simulink model "PMSM_modular_vector_control_sim"  (R2019a)
settings: Solver=ode4  StartTime=0.0  StopTime=Tfinal  FixedStep=Ts  RelTol=1e-3  EnableMultiTasking=on
values from neighbouring files (symbols this model uses):
  Cdc = 150e-6    (= 0.00015)    [PMSM_modular_vector_control_sim_parameters.m]    (also in PMSM_vector_control_single_parameters.m)
  IdPIDmax = Vdcm/5    (= 20)    [PMSM_modular_vector_control_sim_parameters.m]    (also in PMSM_vector_control_single_parameters.m = 54)
  IdPIDmin = -Vdcm/5    (= -20)    [PMSM_modular_vector_control_sim_parameters.m]    (also in PMSM_vector_control_single_parameters.m = -54)
  IdrefM1 = 0    [PMSM_modular_vector_control_sim_parameters.m]
  IdrefM2 = 0    [PMSM_modular_vector_control_sim_parameters.m]
  Inertia = 1e-2    (= 0.01)    [PMSM_modular_vector_control_sim_parameters.m]    (also in PMSM_vector_control_single_parameters.m)
  IqPIDmax = Vdcm-10    (= 90)    [PMSM_modular_vector_control_sim_parameters.m]    (also in PMSM_vector_control_single_parameters.m = 260)
  IqPIDmin = -(Vdcm-10)    (= -90)    [PMSM_modular_vector_control_sim_parameters.m]    (also in PMSM_vector_control_single_parameters.m = -260)
  IrefOverTref = MotorSpeedRad/(EfRated*3)    (= 0.261799387799)    [PMSM_modular_vector_control_sim_parameters.m]    (also in PMSM_vector_control_single_parameters.m)
  LoadTorque1 = 2    [PMSM_modular_vector_control_sim_parameters.m]    (also in PMSM_vector_control_single_parameters.m = 30)
  LoadTorque2 = 2    [PMSM_modular_vector_control_sim_parameters.m]    (also in PMSM_vector_control_single_parameters.m = 20)
  LoadTorqueStepTime = 3    [PMSM_modular_vector_control_sim_parameters.m]    (also in PMSM_vector_control_single_parameters.m = 0.5)
  MechanicalLoadTorque1 = 2    [PMSM_modular_vector_control_sim_parameters.m]
  phase = [0 0 0 0]    [PMSM_modular_vector_control_sim_parameters.m]    (also in PMSM_vector_control_single_parameters.m)
  PMSMLoadResistance = 1e3    (= 1000)    [PMSM_modular_vector_control_sim_parameters.m]
  PolePairs = 10    [PMSM_modular_vector_control_sim_parameters.m]    (also in PMSM_vector_control_single_parameters.m)
  Rin = 1e-3    (= 0.001)    [PMSM_modular_vector_control_sim_parameters.m]    (also in PMSM_vector_control_single_parameters.m)
  Ripth = 0.1    [PMSM_modular_vector_control_sim_parameters.m]    (also in PMSM_vector_control_single_parameters.m)
  Rs = 321e-3    (= 0.321)    [PMSM_modular_vector_control_sim_parameters.m]    (also in PMSM_vector_control_single_parameters.m)
  SpeedPIDmax = 20    [PMSM_modular_vector_control_sim_parameters.m]    (also in PMSM_vector_control_single_parameters.m = 60)
  SpeedPIDmin = -20    [PMSM_modular_vector_control_sim_parameters.m]    (also in PMSM_vector_control_single_parameters.m = -60)
  SpeedRef1 = 200    [PMSM_modular_vector_control_sim_parameters.m]    (also in PMSM_vector_control_single_parameters.m = 600)
  SpeedRef2 = 100    [PMSM_modular_vector_control_sim_parameters.m]    (also in PMSM_vector_control_single_parameters.m = 200)
  SpeedRefStepTime = 6    [PMSM_modular_vector_control_sim_parameters.m]    (also in PMSM_vector_control_single_parameters.m = 0.5)
  Ts = 1000e-9    (= 1e-06)    [PMSM_modular_vector_control_sim_parameters.m]    (also in PMSM_vector_control_single_parameters.m)
  Vdc = 200    [PMSM_modular_vector_control_sim_parameters.m]    (also in PMSM_vector_control_single_parameters.m = 270)
  Vin = Vdc + Rin*(Pout/Vdc)    (= 200.01)    [PMSM_modular_vector_control_sim_parameters.m]    (also in PMSM_vector_control_single_parameters.m = 270.007407407)
  ViscousFriction = 1e-3    (= 0.001)    [PMSM_modular_vector_control_sim_parameters.m]    (also in PMSM_vector_control_single_parameters.m)
undefined symbols (not defined in the file or in its folder): Lload, Rload
libraries: powerlib x41, powerlib_meascontrol x33, fl_lib x12, simulink x9, nesl_utility x8, sdl_lib x2
(part 1 of 2)
settings Model: Creator=ugurm  LastModifiedBy=hakan
settings DataIOCC: LimitDataPoints=on  SaveFormat=Array  ReturnWorkspaceOutputs=off
settings OptimizationCC: LifeSpan=inf
settings DebuggingCC: UnderspecifiedInitializationDetection=Classic  MergeDetectMultiDrivingBlocksExec=none  SolverPrmCheckMsg=warning  StateNameClashWarn=warning  SFUnexpectedBacktrackingDiag=warning  SFNoUnconditionalDefaultTransitionDiag=warning  ArithmeticOperatorsInVariantConditions=warning
settings HardwareCC: ProdBitPerPointer=32  ProdBitPerSizeT=32  ProdBitPerPtrDiffT=32  ProdLargestAtomicFloat=None  ProdIntDivRoundTo=Undefined  ProdEndianess=Unspecified  ProdWordSize=32  ProdHWDeviceType=32-bit Generic
settings ModelReferenceCC: PropagateSignalLabelsOutOfModel=off
settings SFSimCC: SimUseLocalCustomCode=off
settings RTWCC: RTWUseLocalCustomCode=off
settings CodeAppCC: StateflowObjectComments=on
settings GRTTargetCC: TargetLangStandard=C89/C90 (ANSI)  GeneratePreprocessorConditionals=Disable all
settings ConfigComp: CovMetricSettings=dw  CovHtmlReporting=on  CovSaveCumulativeToWorkspaceVar=on  CovSaveSingleToWorkspaceVar=on  CovExternalEMLEnable=off
settings SimscapeCC: SimscapeNormalizeSystem=off

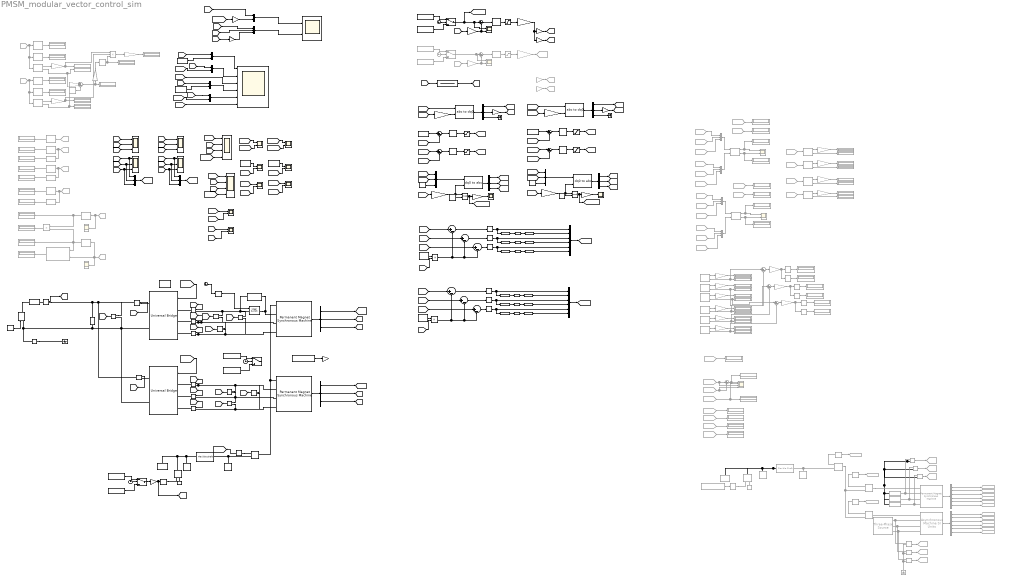
== system PMSM_modular_vector_control_sim ==
  Asynchronous Machine SI Units2 : powerlib/Machines/Asynchronous Machine SI Units  Commented=on  RotorType=Squirrel-cage  PresetModel="16:  10 HP (7.5KW)  400 V 50Hz 1440 RPM"  MechanicalLoad=Mechanical rotational port  ShowDetailedParameters=on  ReferenceFrame=Rotor  Units=SI  MeasurementBus=off  NominalParameters=[7500 400 50]  Stator=[0.7384 0.003045]  Rotor=[0.7402 0.003045]  Cage1=[0.4155 0.002066]  Cage2=[0.4168 0.0003495]  Lm=0.1241  Mechanical=[0.0343 0.000503 2]  PolePairs=2  InitialConditions=[0 0 0 0 0 0 0 0]  SimulateSaturation=off  Saturation=[14.03593122, 27.81365428, 53.79336849, 72.68890987, 97.98006896, 148.6815601, 215.7428561, 302.9841135, 428.7778367 ; 230, 322, 414, 460, 506, 552, 598, 644, 690]  LoadFlowParameters=1492000  TsPowergui=0  TsBlock=-1  IterativeModel=Trapezoidal non iterative  IterativeDiscreteModel=Trapezoidal non iterative  Pmec=1.492e+006
      settings: SourceProductName=Simscape Electrical
  Bus Creator : BusCreator  Inputs=3
  Bus Creator{1..5} (5 alike) : BusCreator  Inputs=2
  Bus Selector : BusSelector  Commented=on  OutputSignals=Mechanical.Rotor speed (wm),Mechanical.Electromagnetic torque Te (N*m),Mechanical.Rotor angle thetam (rad),Stator measurements.Stator current is_a (A),Stator measurements.Stator current is_b (A),Stator measurements.Stator current is_c (A)
  Bus Selector1 : BusSelector  Commented=on  OutputSignals=Rotor speed wm (rad/s),Electromagnetic torque Te (N*m),Rotor angle thetam (rad),Stator current is_a (A),Stator current is_b (A),Stator current is_c (A)
  Bus Selector2 : BusSelector  OutputSignals=Rotor angle thetam (rad),Rotor speed wm (rad/s),Electromagnetic torque Te (N*m)
  Bus Selector3 : BusSelector  OutputSignals=Rotor angle thetam (rad),Rotor speed wm (rad/s),Electromagnetic torque Te (N*m)
  Clock{,1..2,4} (4 alike) : Clock
  Clock3 : Clock  Commented=on
  Compare To Constant : simulink/Logic and Bit Operations/Compare To Constant  relop=<=  const=3.0  OutDataTypeStr=boolean
  Constant1 : Constant  Value=Vin
  Constant10 : Constant  Value=2*pi
  Constant11 : Constant  Value=SpeedRef2
  Constant13 : Constant  Value=LoadTorque2
  Constant16 : Constant  Value=LoadTorque1
  Constant17 : Constant  Commented=on  Value=SpeedRef2
  Constant18 : Constant  Commented=on  Value=SpeedRef1
  Constant19 : Constant  Value=LoadTorque2
  Constant20 : Constant  Value=LoadTorque1
  Constant3 : Constant  Commented=on  Value=-MechanicalLoadTorque1
  Constant4 : Constant  Value=MechanicalLoadTorque1
  Constant5 : Constant  Value=2*pi
  Constant6 : Constant  Value=SpeedRef1
  Constant7 : Constant  Value=0
  Constant8 : Constant  Value=0
  Constant9 : Constant  Commented=on  Value=sqrt(3)
  Current Measurement : powerlib/Measurements/Current Measurement  PhasorSimulation=off  OutputType=Complex  PSBequivalent=0
      settings: SourceProductName=Simscape Electrical
  Current Measurement1 : powerlib/Measurements/Current Measurement  PhasorSimulation=off  OutputType=Complex  PSBequivalent=0
      settings: SourceProductName=Simscape Electrical
  Data Type Conversion{1,3,5,7,9,11} (6 alike) : DataTypeConversion  OutDataTypeStr=boolean
  Data Type Conversion{2,4,6,8,10,12} (6 alike) : DataTypeConversion  OutDataTypeStr=double
  Demux{,1..3} (4 alike) : Demux  Outputs=3
  Display{,1..62} (63 alike) : Display  Commented=on
  Flexible Shaft : sdl_lib/Couplings & Drives/Flexible Shaft  Commented=on  modelTransverse=simscape.enum.onoff.off  parameterization=1  n_segments=10  shaft_stiffness=MechanicalShaftStiffness N*m/rad  shaft_inertia=MechanicalShaftInertia kg*m^2  length=1 m  eiIN=5e5 m^4*Pa  rhoaIN=19 kg/m  shaft_construction=1  diameter_outer=0.075 m  diameter_inner=0.05 m  density=7.8e+3 kg/m^3  shear_modulus=7.93e+10 Pa  elastic_modulus=200e9 Pa  damping_ratio=MechanicalShaftDampingRatio  mu_visc=[ 0 0 ] N*m/(rad/s)  boundaryC=sdl.enum.shaftSupport.clamp  KtransC_row=[10000000, 10000000] N/m  KrotC_row=[10000000, 10000000] N*m/rad  boundaryR=sdl.enum.shaftSupport.clamp  KtransR_row=[10000000, 10000000] N/m  KrotR_row=[10000000, 10000000] N*m/rad  alpha=10 1/s  beta=1e-8 s  d_bearing_trans=[0, 0] N/(m/s)  d_bearing_rotation=[0, 0] N*m/(rad/s)  noDisk=sdl.enum.shaftDisks.none  zDisk=0.5 m  mDiskIN=2 kg  IdDiskIN=0.025 kg*m^2  IpDiskIN=0.050 kg*m^2  offsetMR=[.01, .01] m*kg  offsetMassLocation=[.33, .67] m  offsetMR_initialAngleIN=[0, pi] rad  AnalysisMethod=sdl.enum.bendingAnalysisMethod.LumpedMass  ModeInputMethod=sdl.enum.modeInputMethod.SimscapeDetermined  numModesIn=6  OmegaNom=100 rpm  dw=5 rad/s  dwRefineFactor=1e-4  wMax=50000 rad/s  dz=0.01 m  userMode_w=[162, 162, 649, 649, 1460, 1460, 2596, 2596] rad/s  userMode_z=[0 : 0.1 : 1] m  userMode_shape=[0, 0, 0, 0, 0, 0, 0, 0, 0, 0, 0, 0, 0, 0, 0, 0; .309, 0, 0, .309, .5878, 0, 0, .5878, .809, 0, 0, .809, .9511, 0, 0, .9511; .5878, 0, 0, .5878, .9511, 0, 0, .9511, .9511, 0, 0, .9511, .5878, 0, 0, .5878; .809, 0, 0, .809, .9511, 0, 0, .9511, .309, 0, 0, .309, -.5878, 0, 0, -.5878; .9511, 0, 0, .9511, .5878, 0, 0, .5878, -.5878, 0, 0, -.5878, -.9511, 0, 0, -.9511; 1, 0, 0, 1, 0, 0, 0, 0, -1, 0, 0, -1, 0, 0, 0, 0; .9511, 0, 0, .9511, -.5878, 0, 0, -.5878, -.5878, 0, 0, -.5878, .9511, 0, 0, .9511; .809, 0, 0, .809, -.9511, 0, 0, -.9511, .309, 0, 0, .309, .5878, 0, 0, .5878; .5878, 0, 0, .5878, -.9511, 0, 0, -.9511, .9511, 0, 0, .9511, -.5878, 0, 0, -.5878; .309, 0, 0, .309, -.5878, 0, 0, -.5878, .809, 0, 0, .809, -.9511, 0, 0, -.9511; 0, 0, 0, 0, 0, 0, 0, 0, 0, 0, 0, 0, 0, 0, 0, 0]  initial_deflection=0 rad  initial_velocity=0 rpm
      settings: SourceProductName=Simscape Driveline  SourceProductBaseCode=LD
  Flexible Shaft1 : sdl_lib/Couplings & Drives/Flexible Shaft  modelTransverse=simscape.enum.onoff.off  parameterization=1  n_segments=10  shaft_stiffness=MechanicalShaftStiffness N*m/rad  shaft_inertia=MechanicalShaftInertia kg*m^2  length=1 m  eiIN=5e5 m^4*Pa  rhoaIN=19 kg/m  shaft_construction=1  diameter_outer=0.075 m  diameter_inner=0.05 m  density=7.8e+3 kg/m^3  shear_modulus=7.93e+10 Pa  elastic_modulus=200e9 Pa  damping_ratio=MechanicalShaftDampingRatio  mu_visc=[ 0 0 ] N*m/(rad/s)  boundaryC=sdl.enum.shaftSupport.clamp  KtransC_row=[10000000, 10000000] N/m  KrotC_row=[10000000, 10000000] N*m/rad  boundaryR=sdl.enum.shaftSupport.clamp  KtransR_row=[10000000, 10000000] N/m  KrotR_row=[10000000, 10000000] N*m/rad  alpha=10 1/s  beta=1e-8 s  d_bearing_trans=[0, 0] N/(m/s)  d_bearing_rotation=[0, 0] N*m/(rad/s)  noDisk=sdl.enum.shaftDisks.none  zDisk=0.5 m  mDiskIN=2 kg  IdDiskIN=0.025 kg*m^2  IpDiskIN=0.050 kg*m^2  offsetMR=[.01, .01] m*kg  offsetMassLocation=[.33, .67] m  offsetMR_initialAngleIN=[0, pi] rad  AnalysisMethod=sdl.enum.bendingAnalysisMethod.LumpedMass  ModeInputMethod=sdl.enum.modeInputMethod.SimscapeDetermined  numModesIn=6  OmegaNom=100 rpm  dw=5 rad/s  dwRefineFactor=1e-4  wMax=50000 rad/s  dz=0.01 m  userMode_w=[162, 162, 649, 649, 1460, 1460, 2596, 2596] rad/s  userMode_z=[0 : 0.1 : 1] m  userMode_shape=[0, 0, 0, 0, 0, 0, 0, 0, 0, 0, 0, 0, 0, 0, 0, 0; .309, 0, 0, .309, .5878, 0, 0, .5878, .809, 0, 0, .809, .9511, 0, 0, .9511; .5878, 0, 0, .5878, .9511, 0, 0, .9511, .9511, 0, 0, .9511, .5878, 0, 0, .5878; .809, 0, 0, .809, .9511, 0, 0, .9511, .309, 0, 0, .309, -.5878, 0, 0, -.5878; .9511, 0, 0, .9511, .5878, 0, 0, .5878, -.5878, 0, 0, -.5878, -.9511, 0, 0, -.9511; 1, 0, 0, 1, 0, 0, 0, 0, -1, 0, 0, -1, 0, 0, 0, 0; .9511, 0, 0, .9511, -.5878, 0, 0, -.5878, -.5878, 0, 0, -.5878, .9511, 0, 0, .9511; .809, 0, 0, .809, -.9511, 0, 0, -.9511, .309, 0, 0, .309, .5878, 0, 0, .5878; .5878, 0, 0, .5878, -.9511, 0, 0, -.9511, .9511, 0, 0, .9511, -.5878, 0, 0, -.5878; .309, 0, 0, .309, -.5878, 0, 0, -.5878, .809, 0, 0, .809, -.9511, 0, 0, -.9511; 0, 0, 0, 0, 0, 0, 0, 0, 0, 0, 0, 0, 0, 0, 0, 0]  initial_deflection=0 rad  initial_velocity=0 rpm
      settings: SourceProductName=Simscape Driveline  SourceProductBaseCode=LD
  Fourier1 : powerlib_meascontrol/Measurements/Fourier  Commented=on  Freq=fout  n=1  InInit=[0, 0]  Ts=Ts
      settings: SourceProductName=Simscape Electrical
  Fourier10 : powerlib_meascontrol/Measurements/Fourier  Commented=on  Freq=100  n=1  InInit=[0, 0]  Ts=0
      settings: SourceProductName=Simscape Electrical
  Fourier{3..8,11..12} (8 alike) : powerlib_meascontrol/Measurements/Fourier  Commented=on  Freq=50  n=1  InInit=[0, 0]  Ts=0
      settings: SourceProductName=Simscape Electrical
  Fourier2 : powerlib_meascontrol/Measurements/Fourier  Commented=on  Freq=fout  n=1  InInit=[0, 0]  Ts=Ts
      settings: SourceProductName=Simscape Electrical
  Fourier9 : powerlib_meascontrol/Measurements/Fourier  Commented=on  Freq=100  n=1  InInit=[0, 0]  Ts=0
      settings: SourceProductName=Simscape Electrical
  From : From  Commented=on  GotoTag=Vdc
  From1 : From  Commented=on  GotoTag=Iin
  From12 : From  Commented=on  GotoTag=Isa
  From15 : From  Commented=on  GotoTag=Vab
  From2 : From  Commented=on  GotoTag=Iin
  From3 : From  Commented=on  GotoTag=Idc2
  From30 : From  Commented=on  GotoTag=TorqueM1
  From31 : From  Commented=on  GotoTag=SpeedM1
  From32 : From  Commented=on  GotoTag=TorqueM2
  From33 : From  Commented=on  GotoTag=TorqueM2
  From34 : From  Commented=on  GotoTag=VM2PhA
  From35 : From  Commented=on  GotoTag=TorqueTotal
  From36 : From  Commented=on  GotoTag=TorqueMod1
  From37 : From  Commented=on  GotoTag=TorqueMod2
  From38 : From  Commented=on  GotoTag=TorqueM1
  From39 : From  Commented=on  GotoTag=TorqueM1
  From4 : From  Commented=on  GotoTag=Icap
  From40 : From  Commented=on  GotoTag=VM1PhA
  From41 : From  Commented=on  GotoTag=VM1PhB
  From42 : From  Commented=on  GotoTag=VM1PhC
  From43 : From  Commented=on  GotoTag=IM1PhA
  From44 : From  Commented=on  GotoTag=IM1PhB
  From45 : From  Commented=on  GotoTag=IM1PhC
  From46 : From  Commented=on  GotoTag=VM2PhB
  From47 : From  Commented=on  GotoTag=VM2PhC
  From48 : From  Commented=on  GotoTag=IM2PhA
  From49 : From  Commented=on  GotoTag=IM2PhB
  From5 : From  Commented=on  GotoTag=SpeedM1
  From50 : From  Commented=on  GotoTag=IM2PhC
  From51 : From  Commented=on  GotoTag=SpeedM2
  From52 : From  Commented=on  GotoTag=TorqueM2
  From53 : From  Commented=on  GotoTag=VM1PhA
  From54 : From  Commented=on  GotoTag=IM1PhA
  From55 : From  Commented=on  GotoTag=VM2PhA
  From56 : From  Commented=on  GotoTag=IM2PhA
  From58 : From  Commented=on  GotoTag=Idc1
  From92 : From  Commented=on  GotoTag=wmM2
  Gain{,4,26,28} (4 alike) : Gain  Gain=PolePairs
  Gain{1,9,13..22} (12 alike) : Gain  Commented=on  Gain=1/sqrt(2)
  Gain{6,8,10,12} (4 alike) : Gain  Commented=on  Gain=pi/180
  Gain11 : Gain
  Gain2 : Gain  Gain=30/pi
  Gain23 : Gain  Gain=0.5
  Gain24 : Gain  Gain=0.5
  Gain25 : Gain  Gain=0.5
  Gain27 : Gain
  Gain29 : Gain  Gain=180/pi
  Gain3 : Gain  Gain=IrefOverTref
  Gain30 : Gain  Commented=on  Gain=30/pi
  Gain31 : Gain  Commented=on  Gain=0.5
  Gain32 : Gain  Commented=on  Gain=0.5
  Gain33 : Gain  Commented=on  Gain=IrefOverTref
  Gain34 : Gain  Gain=-2
  Gain35 : Gain  Gain=1/PolePairs
  Gain36 : Gain  Gain=-1
  Gain5 : Gain  Commented=on  Gain=sqrt(3)
  Gain7 : Gain  Gain=180/pi
  Goto2 : Goto  Commented=on  GotoTag=IqrefM2
  Goto24 : Goto  Commented=on  GotoTag=ThetaM2
  Goto25 : Goto  Commented=on  GotoTag=TorqueM2
  Goto26 : Goto  Commented=on  GotoTag=SpeedM2
  Goto27 : Goto  Commented=on  GotoTag=ThetaM1
  Goto28 : Goto  Commented=on  GotoTag=TorqueM1
  Goto29 : Goto  Commented=on  GotoTag=SpeedM1
  Goto30 : Goto  Commented=on  GotoTag=TorqueTotal
  Goto31 : Goto  Commented=on  GotoTag=TorqueMod1
  Goto32 : Goto  Commented=on  GotoTag=TorqueMod2
  Goto33 : Goto  Commented=on  GotoTag=VM1PhA
  Goto34 : Goto  Commented=on  GotoTag=VM1PhB
  Goto35 : Goto  Commented=on  GotoTag=VM1PhC
  Goto36 : Goto  Commented=on  GotoTag=IM1PhC
  Goto37 : Goto  Commented=on  GotoTag=IM1PhB
  Goto38 : Goto  Commented=on  GotoTag=IM1PhA
  Goto39 : Goto  Commented=on  GotoTag=IM2PhC
  Goto40 : Goto  Commented=on  GotoTag=IM2PhB
  Goto41 : Goto  Commented=on  GotoTag=IM2PhA
  Goto42 : Goto  Commented=on  GotoTag=VM2PhA
  Goto43 : Goto  Commented=on  GotoTag=VM2PhB
  Goto44 : Goto  Commented=on  GotoTag=VM2PhC
  Goto69 : Goto  Commented=on  GotoTag=IqrefM1
  Goto70 : Goto  Commented=on  GotoTag=IqrefM2
  Ground1 : powerlib/Elements/Ground  Commented=on  LConnTagsString=a
      settings: SourceProductName=Simscape Electrical
  Ground5 : powerlib/Elements/Ground  LConnTagsString=a
      settings: SourceProductName=Simscape Electrical
  Idc_m{1,3..5,14,16..17} (7 alike) : powerlib/Measurements/Current Measurement  PhasorSimulation=off  OutputType=Complex  PSBequivalent=0
      settings: SourceProductName=Simscape Electrical
  Ideal Switch : powerlib/Power Electronics/Ideal Switch  Ron=0.001  Lon=0  IC=0  Rs=1e5  Cs=inf  Measurements=on
      settings: SourceProductName=Simscape Electrical
  Ideal Torque Sensor1 : fl_lib/Mechanical/Mechanical Sensors/Ideal Torque Sensor  Commented=on
  Ideal Torque Sensor2 : fl_lib/Mechanical/Mechanical Sensors/Ideal Torque Sensor  Commented=on
  Ideal Torque Sensor3 : fl_lib/Mechanical/Mechanical Sensors/Ideal Torque Sensor  Commented=on
  Ideal Torque Sensor5 : fl_lib/Mechanical/Mechanical Sensors/Ideal Torque Sensor
  Ideal Torque Source1 : fl_lib/Mechanical/Mechanical Sources/Ideal Torque Source  Commented=on
  Ideal Torque Source2 : fl_lib/Mechanical/Mechanical Sources/Ideal Torque Source
  Inertia : fl_lib/Mechanical/Rotational Elements/Inertia  Commented=on  inertia=MechanicalInertia1 kg*m^2  w_specify=off  w_priority=High  w=0 rad/s  w_nominal_specify=off  w_nominal_unit=rad/s  w_nominal_value=1  t_specify=off  t_priority=None  t=0 N*m  t_nominal_specify=off  t_nominal_unit=N*m  t_nominal_value=1
  Inertia1 : fl_lib/Mechanical/Rotational Elements/Inertia  Commented=on  inertia=MechanicalInertia1 kg*m^2  w_specify=off  w_priority=High  w=0 rad/s  w_nominal_specify=off  w_nominal_unit=rad/s  w_nominal_value=1  t_specify=off  t_priority=None  t=0 N*m  t_nominal_specify=off  t_nominal_unit=N*m  t_nominal_value=1
  Inertia2 : fl_lib/Mechanical/Rotational Elements/Inertia  inertia=MechanicalInertia1 kg*m^2  w_specify=off  w_priority=High  w=0 rad/s  w_nominal_specify=off  w_nominal_unit=rad/s  w_nominal_value=1  t_specify=off  t_priority=None  t=0 N*m  t_nominal_specify=off  t_nominal_unit=N*m  t_nominal_value=1
  Inertia3 : fl_lib/Mechanical/Rotational Elements/Inertia  inertia=MechanicalInertia1 kg*m^2  w_specify=off  w_priority=High  w=0 rad/s  w_nominal_specify=off  w_nominal_unit=rad/s  w_nominal_value=1  t_specify=off  t_priority=None  t=0 N*m  t_nominal_specify=off  t_nominal_unit=N*m  t_nominal_value=1
  Logical Operator{,1..5} (6 alike) : Logic  Operator=NOT  AllPortsSameDT=off  OutDataTypeStr=boolean
  Math Function : Math  Operator=mod  SaturateOnIntegerOverflow=on
  Math Function1 : Math  Operator=mod  SaturateOnIntegerOverflow=on
  Mean{,1..4} (5 alike) : powerlib_meascontrol/Measurements/Mean  Commented=on  Freq=fout  Vinit=0  Ts=0
      settings: SourceProductName=Simscape Electrical
  Mechanical Rotational Reference : fl_lib/Mechanical/Rotational Elements/Mechanical Rotational Reference  Commented=on
  Mechanical Rotational Reference1 : fl_lib/Mechanical/Rotational Elements/Mechanical Rotational Reference
  Mux{,1,5..6} (4 alike) : Mux  Commented=on  Inputs=3
  Mux{2..3,8..9} (4 alike) : Mux  Inputs=3
  Mux4 : Mux  Inputs=6
  Mux7 : Mux  Inputs=6
  PI iq1 : simulink/Continuous/PID Controller  Controller=PI  Form=Parallel  TimeDomain=Discrete-time  SampleTime=-1  IntegratorMethod=Forward Euler  FilterMethod=Forward Euler  ControllerParametersSource=internal  P=0.1  I=1  D=0  UseFilter=on  N=100  TunerSelectOption=Transfer Function Based (PID Tuner App)  InitialConditionSource=internal  InitialConditionForIntegrator=0  InitialConditionForFilter=0  DifferentiatorICPrevScaledInput=0  ExternalReset=none  TrackingMode=off  Kt=1  LimitOutput=off  UpperSaturationLimit=inf  LowerSaturationLimit=-inf  LinearizeAsGain=on  AntiWindupMode=none  Kb=1  POutMin=[]  POutMax=[]  IOutMin=[]  IOutMax=[]  DOutMin=[]  DOutMax=[]  NOutMin=[]  NOutMax=[]  SumOutMin=[]  SumOutMax=[]  SaturationOutMin=[]  SaturationOutMax=[]  PParamMin=[]  PParamMax=[]  IParamMin=[]  IParamMax=[]  DParamMin=[]  DParamMax=[]  NParamMin=[]  NParamMax=[]  KbParamMin=[]  KbParamMax=[]  KtParamMin=[]  KtParamMax=[]  KbOutMin=[]  KbOutMax=[]  KtOutMin=[]  KtOutMax=[]  IntegratorOutMin=[]  IntegratorOutMax=[]  FilterOutMin=[]  FilterOutMax=[]  SumI1OutMin=[]  SumI1OutMax=[]  SumI2OutMin=[]  SumI2OutMax=[]  SumI3OutMin=[]  SumI3OutMax=[]  SumI4OutMin=[]  SumI4OutMax=[]  SumDOutMin=[]  SumDOutMax=[]  DifferentiatorOutMin=[]  DifferentiatorOutMax=[]  FilterDiffOutCoefMin=[]  FilterDiffOutCoefMax=[]  ReciprocalOutMin=[]  ReciprocalOutMax=[]  SumDenOutMin=[]  SumDenOutMax=[]  SumNumOutMin=[]  SumNumOutMax=[]  DivideOutMin=[]  DivideOutMax=[]  IntegratorContinuousStateAttributes=''  IntegratorStateMustResolveToSignalObject=off  IntegratorRTWStateStorageClass=Auto  FilterContinuousStateAttributes=''  FilterStateMustResolveToSignalObject=off  FilterRTWStateStorageClass=Auto  ParallelPVariant=InternalParameters  IdealPVariant=Disabled  IVariant=InternalParameters  DVariant=Disabled  IntegratorVariant=Discrete  SatVariant=Disabled  AWVariant=Passthrough  PCopyVariant=Disabled  TRVariant=Disabled  FdbkBlocksVariant=Forward  IdealPFdbkVariant=Disabled  SatFdbkVariant=Disabled  DerivativeFilterVariant=Disabled  NVariant=Disabled  NCopyVariant=Disabled_SignalSpec  FilterICVariant=Disabled  IntegratorICVariant=InternalICs  ExternalResetVariant=Disabled  TRSumVariant=Passthrough  SumFdbkVariant=Disabled  SumVariant=Sum_PI
  PI iq{2..5} (4 alike) : simulink/Continuous/PID Controller  Controller=PI  Form=Parallel  TimeDomain=Discrete-time  SampleTime=-1  IntegratorMethod=Forward Euler  FilterMethod=Forward Euler  ControllerParametersSource=internal  P=100  I=100  D=0  UseFilter=on  N=100  TunerSelectOption=Transfer Function Based (PID Tuner App)  InitialConditionSource=internal  InitialConditionForIntegrator=0  InitialConditionForFilter=0  DifferentiatorICPrevScaledInput=0  ExternalReset=none  TrackingMode=off  Kt=1  LimitOutput=off  UpperSaturationLimit=inf  LowerSaturationLimit=-inf  LinearizeAsGain=on  AntiWindupMode=none  Kb=1  POutMin=[]  POutMax=[]  IOutMin=[]  IOutMax=[]  DOutMin=[]  DOutMax=[]  NOutMin=[]  NOutMax=[]  SumOutMin=[]  SumOutMax=[]  SaturationOutMin=[]  SaturationOutMax=[]  PParamMin=[]  PParamMax=[]  IParamMin=[]  IParamMax=[]  DParamMin=[]  DParamMax=[]  NParamMin=[]  NParamMax=[]  KbParamMin=[]  KbParamMax=[]  KtParamMin=[]  KtParamMax=[]  KbOutMin=[]  KbOutMax=[]  KtOutMin=[]  KtOutMax=[]  IntegratorOutMin=[]  IntegratorOutMax=[]  FilterOutMin=[]  FilterOutMax=[]  SumI1OutMin=[]  SumI1OutMax=[]  SumI2OutMin=[]  SumI2OutMax=[]  SumI3OutMin=[]  SumI3OutMax=[]  SumI4OutMin=[]  SumI4OutMax=[]  SumDOutMin=[]  SumDOutMax=[]  DifferentiatorOutMin=[]  DifferentiatorOutMax=[]  FilterDiffOutCoefMin=[]  FilterDiffOutCoefMax=[]  ReciprocalOutMin=[]  ReciprocalOutMax=[]  SumDenOutMin=[]  SumDenOutMax=[]  SumNumOutMin=[]  SumNumOutMax=[]  DivideOutMin=[]  DivideOutMax=[]  IntegratorContinuousStateAttributes=''  IntegratorStateMustResolveToSignalObject=off  IntegratorRTWStateStorageClass=Auto  FilterContinuousStateAttributes=''  FilterStateMustResolveToSignalObject=off  FilterRTWStateStorageClass=Auto  ParallelPVariant=InternalParameters  IdealPVariant=Disabled  IVariant=InternalParameters  DVariant=Disabled  IntegratorVariant=Discrete  SatVariant=Disabled  AWVariant=Passthrough  PCopyVariant=Disabled  TRVariant=Disabled  FdbkBlocksVariant=Forward  IdealPFdbkVariant=Disabled  SatFdbkVariant=Disabled  DerivativeFilterVariant=Disabled  NVariant=Disabled  NCopyVariant=Disabled_SignalSpec  FilterICVariant=Disabled  IntegratorICVariant=InternalICs  ExternalResetVariant=Disabled  TRSumVariant=Passthrough  SumFdbkVariant=Disabled  SumVariant=Sum_PI
  PI iq6 : simulink/Continuous/PID Controller  Commented=on  Controller=PI  Form=Parallel  TimeDomain=Discrete-time  SampleTime=-1  IntegratorMethod=Forward Euler  FilterMethod=Forward Euler  ControllerParametersSource=internal  P=0.1  I=1  D=0  UseFilter=on  N=100  TunerSelectOption=Transfer Function Based (PID Tuner App)  InitialConditionSource=internal  InitialConditionForIntegrator=0  InitialConditionForFilter=0  DifferentiatorICPrevScaledInput=0  ExternalReset=none  TrackingMode=off  Kt=1  LimitOutput=off  UpperSaturationLimit=inf  LowerSaturationLimit=-inf  LinearizeAsGain=on  AntiWindupMode=none  Kb=1  POutMin=[]  POutMax=[]  IOutMin=[]  IOutMax=[]  DOutMin=[]  DOutMax=[]  NOutMin=[]  NOutMax=[]  SumOutMin=[]  SumOutMax=[]  SaturationOutMin=[]  SaturationOutMax=[]  PParamMin=[]  PParamMax=[]  IParamMin=[]  IParamMax=[]  DParamMin=[]  DParamMax=[]  NParamMin=[]  NParamMax=[]  KbParamMin=[]  KbParamMax=[]  KtParamMin=[]  KtParamMax=[]  KbOutMin=[]  KbOutMax=[]  KtOutMin=[]  KtOutMax=[]  IntegratorOutMin=[]  IntegratorOutMax=[]  FilterOutMin=[]  FilterOutMax=[]  SumI1OutMin=[]  SumI1OutMax=[]  SumI2OutMin=[]  SumI2OutMax=[]  SumI3OutMin=[]  SumI3OutMax=[]  SumI4OutMin=[]  SumI4OutMax=[]  SumDOutMin=[]  SumDOutMax=[]  DifferentiatorOutMin=[]  DifferentiatorOutMax=[]  FilterDiffOutCoefMin=[]  FilterDiffOutCoefMax=[]  ReciprocalOutMin=[]  ReciprocalOutMax=[]  SumDenOutMin=[]  SumDenOutMax=[]  SumNumOutMin=[]  SumNumOutMax=[]  DivideOutMin=[]  DivideOutMax=[]  IntegratorContinuousStateAttributes=''  IntegratorStateMustResolveToSignalObject=off  IntegratorRTWStateStorageClass=Auto  FilterContinuousStateAttributes=''  FilterStateMustResolveToSignalObject=off  FilterRTWStateStorageClass=Auto  ParallelPVariant=InternalParameters  IdealPVariant=Disabled  IVariant=InternalParameters  DVariant=Disabled  IntegratorVariant=Discrete  SatVariant=Disabled  AWVariant=Passthrough  PCopyVariant=Disabled  TRVariant=Disabled  FdbkBlocksVariant=Forward  IdealPFdbkVariant=Disabled  SatFdbkVariant=Disabled  DerivativeFilterVariant=Disabled  NVariant=Disabled  NCopyVariant=Disabled_SignalSpec  FilterICVariant=Disabled  IntegratorICVariant=InternalICs  ExternalResetVariant=Disabled  TRSumVariant=Passthrough  SumFdbkVariant=Disabled  SumVariant=Sum_PI
  PS-Simulink Converter1 : nesl_utility/PS-Simulink Converter  Commented=on  PhysicalDomain=network_engine_domain  SubClassName=ps_output  LeftPortType=input  RightPortType=output  PseudoPeriodic=off  Frequencies=[]  Unit=1  AffineConversion=off
  PS-Simulink Converter2 : nesl_utility/PS-Simulink Converter  Commented=on  PhysicalDomain=network_engine_domain  SubClassName=ps_output  LeftPortType=input  RightPortType=output  PseudoPeriodic=off  Frequencies=[]  Unit=1  AffineConversion=off
  PS-Simulink Converter3 : nesl_utility/PS-Simulink Converter  Commented=on  PhysicalDomain=network_engine_domain  SubClassName=ps_output  LeftPortType=input  RightPortType=output  PseudoPeriodic=off  Frequencies=[]  Unit=1  AffineConversion=off
  PS-Simulink Converter5 : nesl_utility/PS-Simulink Converter  PhysicalDomain=network_engine_domain  SubClassName=ps_output  LeftPortType=input  RightPortType=output  PseudoPeriodic=off  Frequencies=[]  Unit=1  AffineConversion=off
  Permanent Magnet Synchronous Machine : powerlib/Machines/Permanent Magnet Synchronous Machine  NbPhases=3  FluxDistribution=Sinusoidal  RotorType=Round  MechanicalLoad=Mechanical rotational port  PresetModel=No  ShowDetailedParameters=on  MeasurementBus=off  Resistance=Rs  Inductance=8.5e-3  dqInductances=[3.1e-3,3.6e-3]  La=Ls  MachineConstant=Voltage Constant (V_peak L-L / krpm)  Flux=0.18006  VoltageCst=VoltageConstant  TorqueCst=2.7009  Flat=120  Mechanical=[Inertia ViscousFriction PolePairs 0]  PolePairs=4  InitialConditions=[0,0, 0,0]  InitialConditions5ph=[0 0 0 0 0 0]  TsPowergui=0  TsBlock=-1  RefAngle=90 degrees behind phase A axis (modified Park)
  Permanent Magnet Synchronous Machine1 : powerlib/Machines/Permanent Magnet Synchronous Machine  Commented=on  NbPhases=3  FluxDistribution=Sinusoidal  RotorType=Round  MechanicalLoad=Mechanical rotational port  PresetModel="07:  20 Nm 300 Vdc 2200 RPM - 33.9 Nm"  ShowDetailedParameters=on  MeasurementBus=off  Resistance=0.129  Inductance=8.5e-3  dqInductances=[3.1e-3,3.6e-3]  La=0.00153  MachineConstant=Flux linkage established by magnets (V.s)  Flux=0.1821  VoltageCst=132.1171  TorqueCst=1.0926  Flat=120  Mechanical=[0.003334 0.000425 4 0]  PolePairs=4  InitialConditions=[0,0, 0,0]  InitialConditions5ph=[0 0 0 0 0 0]  TsPowergui=0  TsBlock=-1  RefAngle=90 degrees behind phase A axis (modified Park)
  Permanent Magnet Synchronous Machine2 : powerlib/Machines/Permanent Magnet Synchronous Machine  NbPhases=3  FluxDistribution=Sinusoidal  RotorType=Round  MechanicalLoad=Mechanical rotational port  PresetModel=No  ShowDetailedParameters=on  MeasurementBus=off  Resistance=Rs  Inductance=8.5e-3  dqInductances=[3.1e-3,3.6e-3]  La=Ls  MachineConstant=Voltage Constant (V_peak L-L / krpm)  Flux=0.18006  VoltageCst=VoltageConstant  TorqueCst=2.7009  Flat=120  Mechanical=[Inertia ViscousFriction PolePairs 0]  PolePairs=4  InitialConditions=[0,0, 0,0]  InitialConditions5ph=[0 0 0 0 0 0]  TsPowergui=0  TsBlock=-1  RefAngle=90 degrees behind phase A axis (modified Park)
  "Power (3ph, Instantaneous)" : powerlib_meascontrol/Measurements/Power (3ph, Instantaneous)  Commented=on
      settings: SourceProductName=Simscape Electrical
  "Power (3ph, Instantaneous)1" : powerlib_meascontrol/Measurements/Power (3ph, Instantaneous)  Commented=on
      settings: SourceProductName=Simscape Electrical
  Product : Product  Commented=on
  Product1 : Product
  Product2 : Product  Commented=on  Inputs=3
  Product3 : Product
  RMS{1..6} (6 alike) : powerlib_meascontrol/Measurements/RMS  Commented=on  TrueRMS=on  Freq=fout  RMSInit=0  Ts=0
      settings: SourceProductName=Simscape Electrical
  Relay{,1..5} (6 alike) : Relay
  Saturation : Saturate  UpperLimit=SpeedPIDmax  LowerLimit=SpeedPIDmin
  Saturation1 : Saturate  UpperLimit=IdPIDmax  LowerLimit=IdPIDmin
  Saturation2 : Saturate  UpperLimit=IqPIDmax  LowerLimit=IqPIDmin
  Saturation3 : Saturate  UpperLimit=IdPIDmax  LowerLimit=IdPIDmin
  Saturation4 : Saturate  UpperLimit=IqPIDmax  LowerLimit=IqPIDmin
  Saturation5 : Saturate  Commented=on  UpperLimit=SpeedPIDmax  LowerLimit=SpeedPIDmin
  Scope1 : Scope  Commented=on
  Scope11 : Scope  Commented=on  NumInputPorts=2
  Scope12 : Scope  Commented=on  NumInputPorts=4
  Scope16 : Scope
  Scope{2,8,17..18} (4 alike) : Scope  NumInputPorts=3
  Scope{9,19..20,22..26,28} (9 alike) : Scope  NumInputPorts=2
  Scope21 : Scope  NumInputPorts=4
  Scope27 : Scope  NumInputPorts=6
  Scope3 : Scope  Commented=on
  Scope5 : Scope  Commented=on  NumInputPorts=2
  Scope6 : Scope
  Scope7 : Scope  NumInputPorts=4
  Series RLC Branch : powerlib/Elements/Series RLC Branch  Commented=on  LConnTagsString=__new0  RConnTagsString=__new0  BranchType=R  Resistance=PMSMLoadResistance  Inductance=1e-3  SetiL0=off  InitialCurrent=0  Capacitance=1e-6  Setx0=off  InitialVoltage=0  Measurements=None
      settings: SourceProductName=Simscape Electrical
  Series RLC Branch1 : powerlib/Elements/Series RLC Branch  Commented=on  LConnTagsString=__new0  RConnTagsString=__new0  BranchType=R  Resistance=PMSMLoadResistance  Inductance=1e-3  SetiL0=off  InitialCurrent=0  Capacitance=1e-6  Setx0=off  InitialVoltage=0  Measurements=None
      settings: SourceProductName=Simscape Electrical
  Series RLC Branch2 : powerlib/Elements/Series RLC Branch  Commented=on  LConnTagsString=__new0  RConnTagsString=__new0  BranchType=R  Resistance=PMSMLoadResistance  Inductance=1e-3  SetiL0=off  InitialCurrent=0  Capacitance=1e-6  Setx0=off  InitialVoltage=0  Measurements=None
      settings: SourceProductName=Simscape Electrical
  Series RLC Branch20 : powerlib/Elements/Series RLC Branch  LConnTagsString=__new0  RConnTagsString=__new0  BranchType=R  Resistance=Rin  Inductance=1e-3  SetiL0=off  InitialCurrent=0  Capacitance=1e-6  Setx0=off  InitialVoltage=0  Measurements=None
      settings: SourceProductName=Simscape Electrical
  Series RLC Branch21 : powerlib/Elements/Series RLC Branch  LConnTagsString=__new0  RConnTagsString=__new0  BranchType=C  Resistance=Rload  Inductance=Lload  SetiL0=off  InitialCurrent=0  Capacitance=Cdc  Setx0=off  InitialVoltage=0  Measurements=None
      settings: SourceProductName=Simscape Electrical
  Series RLC Branch3 : powerlib/Elements/Series RLC Branch  LConnTagsString=__new0  RConnTagsString=__new0  BranchType=R  Resistance=5000  Inductance=1e-3  SetiL0=off  InitialCurrent=0  Capacitance=1e-6  Setx0=off  InitialVoltage=0  Measurements=None
      settings: SourceProductName=Simscape Electrical
  Series RLC Branch40 : powerlib/Elements/Series RLC Branch  LConnTagsString=__new0  RConnTagsString=__new0  BranchType=R  Resistance=1e12  Inductance=Lload  SetiL0=off  InitialCurrent=0  Capacitance=1e-6  Setx0=off  InitialVoltage=0  Measurements=None
      settings: SourceProductName=Simscape Electrical
  Simulink-PS Converter1 : nesl_utility/Simulink-PS Converter  Commented=on  PhysicalDomain=network_engine_domain  SubClassName=ps_input  LeftPortType=input  RightPortType=output  PseudoPeriodic=off  Frequencies=[]  NoiseDistribution=none  NoiseParameters=[]  Unit=1  AffineConversion=off  FilteringAndDerivatives=zero  SimscapeFilterOrder=1  InputFilterTimeConstant=0.001  UdotUserProvided=1
  Simulink-PS Converter2 : nesl_utility/Simulink-PS Converter  PhysicalDomain=network_engine_domain  SubClassName=ps_input  LeftPortType=input  RightPortType=output  PseudoPeriodic=off  Frequencies=[]  NoiseDistribution=none  NoiseParameters=[]  Unit=1  AffineConversion=off  FilteringAndDerivatives=zero  SimscapeFilterOrder=1  InputFilterTimeConstant=0.001  UdotUserProvided=1
  Solver Configuration : nesl_utility/Solver Configuration  Commented=on  PhysicalDomain=network_engine_domain  SubClassName=solver  LeftPortType=input  RightPortType=generic  Tones=[]  Harmonics=[]  SimulateNoise=off  Profile=off  UseLocalSampling=off  EnableSwitchedLinearOptims=on  FrequencyDomain=off  UseCCode=off  RelTol=0.001  AbsTol=1e-06  MinStep=1e-09  ToWorkspace=off  RevertToSquareIcSolve=off  NumHomotopyIterations=100  PhasorMode=off  PhasorModeNumHarmonics=1  DoDC=off  ResidualTolerance=1e-09  UseLocalSolver=off  LocalSolverChoice=NE_BACKWARD_EULER_ADVANCER  LocalSolverSampleTime=0.001  DoFixedCost=off  MaxNonlinIter=3  MaxModeIter=2  LinearAlgebra=Sparse  EquationFormulation=NE_TIME_EF  DelaysMemoryBudget=1024  AutomaticFiltering=on  FilteringTimeConstant=0.001  PartitionStorageMethod=AS_NEEDED  PartitionMemoryBudget=1024  PartitionMethod=FAST
  Solver Configuration1 : nesl_utility/Solver Configuration  PhysicalDomain=network_engine_domain  SubClassName=solver  LeftPortType=input  RightPortType=generic  Tones=[]  Harmonics=[]  SimulateNoise=off  Profile=off  UseLocalSampling=off  EnableSwitchedLinearOptims=on  FrequencyDomain=off  UseCCode=off  RelTol=0.001  AbsTol=1e-06  MinStep=1e-09  ToWorkspace=off  RevertToSquareIcSolve=off  NumHomotopyIterations=100  PhasorMode=off  PhasorModeNumHarmonics=1  DoDC=off  ResidualTolerance=1e-09  UseLocalSolver=off  LocalSolverChoice=NE_BACKWARD_EULER_ADVANCER  LocalSolverSampleTime=0.001  DoFixedCost=off  MaxNonlinIter=3  MaxModeIter=2  LinearAlgebra=Sparse  EquationFormulation=NE_TIME_EF  DelaysMemoryBudget=1024  AutomaticFiltering=on  FilteringTimeConstant=0.001  PartitionStorageMethod=AS_NEEDED  PartitionMemoryBudget=1024  PartitionMethod=FAST
  Subsystem5 : Subsystem  Commented=on
  Sum{,1..5,11..15} (11 alike) : Sum  Inputs=|+-
  Sum{8..10,16} (4 alike) : Sum  Commented=on  Inputs=|+-
  Sum6 : Sum  Commented=on  Inputs=|+--
  Sum7 : Sum  Commented=on  Inputs=|++
  Switch : Switch  Criteria=u2 > Threshold  Threshold=SpeedRefStepTime
  Switch2 : Switch  Criteria=u2 > Threshold  Threshold=LoadTorqueStepTime
  Switch3 : Switch  Commented=on  Criteria=u2 > Threshold  Threshold=SpeedRefStepTime
  Switch4 : Switch  Criteria=u2 > Threshold  Threshold=LoadTorqueStepTime
  THD : powerlib_meascontrol/Measurements/THD  Commented=on  Freq=50  Ts=0
      settings: SourceProductName=Simscape Electrical
  THD1 : powerlib_meascontrol/Measurements/THD  Commented=on  Freq=50  Ts=0
      settings: SourceProductName=Simscape Electrical
  Terminator : Terminator
  Terminator1 : Terminator
  Three-Phase Source : powerlib/Electrical Sources/Three-Phase Source  Commented=on  InternalConnection=Yg  VoltagePhases=off  Voltage=400  PhaseAngle=0  Voltage_phases=[25e3 25e3 25e3]/sqrt(3)  PhaseAngles_phases=[0 -120 +120]  Frequency=50  NonIdealSource=off  SpecifyImpedance=off  Resistance=0.8929  Inductance=16.58e-3  ShortCircuitLevel=100e6  BaseVoltage=25e3  XRratio=7  BusType=swing  Pref=10e3  Qref=0  Prefabc=[10e3, 10e3, 10e3]  Qrefabc=[0, 0, 0]  Qmin=-inf  Qmax=inf
      settings: SourceProductName=Simscape Electrical
  Transfer Fcn : TransferFcn  Denominator=[1/(2*pi*50) 1]
  Triangle Generator : powerlib_meascontrol/Pulse & Signal Generators/Triangle Generator  Freq=fsw  Phase=phase(1)  Ts=Ts
      settings: SourceProductName=Simscape Electrical
  Triangle Generator1 : powerlib_meascontrol/Pulse & Signal Generators/Triangle Generator  Freq=fsw  Phase=phase(2)  Ts=Ts
      settings: SourceProductName=Simscape Electrical
  Trigonometric Function{,1..2,5} (4 alike) : Trigonometry  Commented=on  Operator=cos
  Trigonometric Function3 : Trigonometry  Commented=on
  Trigonometric Function4 : Trigonometry  Commented=on
  Trigonometric Function6 : Trigonometry  Commented=on
  Universal Bridge1 : powerlib/Power Electronics/Universal Bridge  Arms=3  SnubberResistance=1e5  SnubberCapacitance=inf  Device=IGBT / Diodes  Ron=1e-6  Lon=0  ForwardVoltages="[  0  0  ]"  ForwardVoltage=0  GTOparameters=[ 10e-6 , 20e-6 ]  IGBTparameters=[0,0]  Measurements=None  Measurements_2=None  converterType=Rectifier
      settings: SourceProductName=Simscape Electrical
  Universal Bridge4 : powerlib/Power Electronics/Universal Bridge  Arms=3  SnubberResistance=1e5  SnubberCapacitance=inf  Device=IGBT / Diodes  Ron=1e-6  Lon=0  ForwardVoltages="[  0  0  ]"  ForwardVoltage=0  GTOparameters=[ 10e-6 , 20e-6 ]  IGBTparameters=[0,0]  Measurements=None  Measurements_2=None  converterType=Rectifier
      settings: SourceProductName=Simscape Electrical
  Vdc1 : powerlib/Electrical Sources/Controlled Voltage Source  Initialize=off  Source_Type=DC  Amplitude=200  Phase=0  Frequency=0  Measurements=None
      settings: SourceProductName=Simscape Electrical
  Vdc_m{2..7} (6 alike) : powerlib/Measurements/Voltage Measurement  PhasorSimulation=off  OutputType=Complex  PSBequivalent=0
      settings: SourceProductName=Simscape Electrical
  Voltage Measurement{,1..5} (6 alike) : powerlib/Measurements/Voltage Measurement  Commented=on  PhasorSimulation=off  OutputType=Complex  PSBequivalent=0
      settings: SourceProductName=Simscape Electrical
  Voltage Measurement6 : powerlib/Measurements/Voltage Measurement  PhasorSimulation=off  OutputType=Complex  PSBequivalent=0
      settings: SourceProductName=Simscape Electrical
  abc to dq0 : powerlib_meascontrol/Transformations/abc to dq0  Alignment=90 degrees behind phase A axis
      settings: SourceProductName=Simscape Electrical
  abc to dq1 : powerlib_meascontrol/Transformations/abc to dq0  Alignment=90 degrees behind phase A axis
      settings: SourceProductName=Simscape Electrical
  dq0 to abc : powerlib_meascontrol/Transformations/dq0 to abc  Alignment=90 degrees behind phase A axis
      settings: SourceProductName=Simscape Electrical
  dq0 to abc1 : powerlib_meascontrol/Transformations/dq0 to abc  Alignment=90 degrees behind phase A axis
      settings: SourceProductName=Simscape Electrical
  idref : Constant  Value=IdrefM1
  idref1 : Constant  Value=IdrefM1
  idref2 : Constant  Value=IdrefM1
  idref3 : Constant  Value=IdrefM2
  idref4 : Constant  Value=IdrefM2
  idref5 : Constant  Value=IdrefM2
  powergui1 : powerlib/powergui  Priority=1  SimulationMode=Discrete  SampleTime=Ts  frequency=60  Iterations=50  frequencyindice=0  Pbase=100e6  ErrMax=1e-4  UnitsV=kV  UnitsW=MW  buscounter=0  FunctionMessages=off  echomessages=off  EnableUseOfTLC=off  CurrentSourceSwitches=off  DisableSnubberDevices=off  DisableRonSwitches=off  DisableVfSwitches=off  DisplayEquations=off  AutomaticDiscreteSolvers=off  SolverType=Tustin  Interpol=off  ExternalGateDelay=off  methode=off  Ts=0  x0status=blocks  SPID=off  SwTol=0  HookPort=off  NonlinearTolerance=0  nMaxIteration=15  ContinueOnMaxIteration=off  RestoreLinks=warning  ResistiveCurrentMeasurement=off  Frange=[0:2:500]  Ylog=off  Xlog=on  ShowGrid=off  save=off  variable=ZData  structure=Icap  ZoomFFT=off  StartTime=0.04  cycles=5  DisplayStyle=3  fundamental=150  FreqAxis=off  MaxFrequency=1000  frequencyindicesteady=1  RmsSteady=1  display=off
      settings: SourceProductName=Simscape Electrical
  speed : Scope  NumInputPorts=2
  speed1 : Scope  Commented=on  NumInputPorts=2
  wires:
  Idc_m14/1 -> [IsaM1]
  Constant1/1 -> Vdc1/1
  Idc_m16/1 -> [IsbM1]
  Idc_m17/1 -> [IscM1]
  Mean/1 -> Product/2, Subsystem5/1(Vdcavg), Display8/1
  RMS2/1 -> Display4/1
  Current Measurement1/1 -> [Idc1]
  Mean3/1 -> Display7/1
  Subsystem5/1(Out1) -> Display14/1
  Product/1 -> Display17/1
  From/1 -> Scope3/1, Mean/1, Subsystem5/2(vdc)
  Mean1/1 -> Display1/1
  RMS1/1 -> Display2/1
  Fourier1/1 -> Gain9/1
  THD/1 -> Display3/1
  RMS4/1 -> Display5/1
  Gain9/1 -> Product2/1, Display6/1
  Fourier1/2 -> Sum6/2, Display9/1
  Voltage Measurement6/1 -> [Vdc]
  Current Measurement/1 -> [Iin]
  Mean2/1 -> Product/1, Display10/1
  From1/1 -> Scope1/1, Mean2/1
  From2/1 -> Mean1/1, RMS1/1
  From3/1 -> Mean3/1, RMS2/1
  From4/1 -> RMS5/1
  RMS5/1 -> Display11/1
  Vdc_m5/1 -> [VabM1]
  Vdc_m3/1 -> [VbcM1]
  Vdc_m2/1 -> [VcaM1]
  [IsaM1] -> Mux2/1, Scope8/1
  [IsbM1] -> Mux2/2, Scope8/2
  [IscM1] -> Mux2/3, Scope8/3
  [VabM1] -> Scope2/1
  [VbcM1] -> Scope2/2
  [VcaM1] -> Scope2/3
  From12/1 -> Fourier1/1, RMS4/1, THD/1
  THD1/1 -> Display12/1
  RMS3/1 -> Display13/1
  From15/1 -> Fourier2/1, RMS3/1, THD1/1
  Permanent Magnet Synchronous Machine/1 -> Bus Selector3/1
  Bus Selector3/3 -> [TeM1]  "<Electromagnetic torque Te (N*m)>"
  Bus Selector3/2 -> [wmM1]  "<Rotor speed wm (rad/s)>"
  Bus Selector3/1 -> [ThetamM1]  "<Rotor angle thetam (rad)>"
  Mux2/1 -> [IsabcM1]
  [IsabcM1] -> abc to dq0/1
  Gain/1 -> abc to dq0/2
  [ThetamM1] -> Gain/1
  abc to dq0/1 -> Demux/1
  Demux/1 -> [idM1]  "id"
  Demux/2 -> Gain11/1  "iq"
  Demux/3 -> Terminator/1  "i0"
  Fourier2/1 -> Gain1/1
  Gain1/1 -> Product2/2, Display15/1
  Fourier2/2 -> Sum6/1, Display16/1
  [wmM1] -> Gain2/1
  Gain2/1 -> speed/2, Sum1/2
  Switch/1 -> [SpeedRef], Sum1/1, speed/1
  Sum1/1 -> PI iq1/1
  PI iq1/1 -> Saturation/1
  Saturation/1 -> Gain3/1
  [idM1] -> Sum2/2
  Sum2/1 -> PI iq2/1
  PI iq2/1 -> Saturation1/1
  idref/1 -> Sum2/1
  [iqM1] -> Sum3/2
  Sum3/1 -> PI iq3/1
  PI iq3/1 -> Saturation2/1
  [IqrefM1] -> Sum3/1
  Saturation2/1 -> [VqrefM1]
  [ThetamM1] -> Gain4/1
  Gain4/1 -> Math Function/1, dq0 to abc/2
  Constant7/1 -> Mux3/3
  Mux3/1 -> dq0 to abc/1
  [Vdc] -> Transfer Fcn/1
  Transfer Fcn/1 -> [VdcFilt]
  dq0 to abc/1 -> Demux1/1
  Sum/1 -> Relay/1
  Sum4/1 -> Relay1/1
  Sum5/1 -> Relay2/1
  Data Type Conversion1/1 -> Logical Operator/1
  Logical Operator/1 -> Data Type Conversion2/1
  Data Type Conversion2/1 -> Mux4/2
  Data Type Conversion3/1 -> Logical Operator1/1
  Relay1/1 -> Data Type Conversion3/1, Mux4/3
  Logical Operator1/1 -> Data Type Conversion4/1
  Data Type Conversion4/1 -> Mux4/4
  Data Type Conversion5/1 -> Logical Operator2/1
  Relay2/1 -> Data Type Conversion5/1, Mux4/5
  Logical Operator2/1 -> Data Type Conversion6/1
  Data Type Conversion6/1 -> Mux4/6
  Relay/1 -> Mux4/1, Data Type Conversion1/1
  [VmodCM1] -> Sum5/1
  Triangle Generator/1 -> Product1/1
  [VdcFilt] -> Product1/2
  Demux1/1 -> [VmodAM1]
  Demux1/2 -> [VmodBM1]
  Demux1/3 -> [VmodCM1]
  Mux4/1 -> [GateSignalsM1]
  [GateSignalsM1] -> Universal Bridge4/1
  Product1/1 -> Sum/2, Sum4/2, Sum5/2
  Constant9/1 -> Sum6/3
  Sum6/1 -> Display18/1, Gain6/1
  Trigonometric Function/1 -> Display21/1, Product2/3
  Gain6/1 -> Trigonometric Function/1
  Product2/1 -> Gain5/1
  Gain5/1 -> Display19/1
  Constant10/1 -> Math Function/2
  Math Function/1 -> [ThetamModM1], Gain7/1
  Gain7/1 -> Scope6/1
  [IsabcM1] -> Scope7/1
  Gain11/1 -> [iqM1]
  Saturation1/1 -> [VdrefM1]
  [VqrefM1] -> Mux3/2
  [VdrefM1] -> Mux3/1
  Clock/1 -> Switch/2
  Constant11/1 -> Switch/1
  Constant6/1 -> Switch/3
  [VmodAM1] -> Sum/1
  [VmodBM1] -> Sum4/1
  Constant3/1 -> Simulink-PS Converter1/1
  PS-Simulink Converter1/1 -> Goto30/1
  Asynchronous Machine SI Units2/1 -> Bus Selector/1
  Permanent Magnet Synchronous Machine1/1 -> Bus Selector1/1
  Bus Selector/3 -> Goto24/1  "<Rotor angle thetam (rad)>"
  Bus Selector/2 -> Goto25/1  "<Electromagnetic torque Te (N*m)>"
  Bus Selector/1 -> Goto26/1  "<Rotor speed (wm)>"
  Bus Selector1/3 -> Goto27/1  "<Rotor angle thetam (rad)>"
  Bus Selector1/2 -> Goto28/1  "<Electromagnetic torque Te (N*m)>"
  Bus Selector1/1 -> Goto29/1  "<Rotor speed wm (rad/s)>"
  From30/1 -> Scope12/3, Sum7/1
  From33/1 -> Scope12/4, Sum7/2
  Sum7/1 -> Display25/1, Scope12/1
  From35/1 -> Display24/1, Scope12/2
  From31/1 -> Display41/1
  PS-Simulink Converter2/1 -> Goto31/1
  PS-Simulink Converter3/1 -> Goto32/1
  From36/1 -> Display/1
  From38/1 -> Display20/1
  From37/1 -> Display22/1
  From39/1 -> Display23/1
  From40/1 -> Mux/1
  Fourier3/1 -> Gain13/1
  Fourier3/2 -> Sum8/1, Display27/1
  Fourier4/2 -> Sum9/1, Display29/1
  Fourier5/1 -> Gain15/1
  Fourier5/2 -> Sum10/1, Display31/1
  From42/1 -> Mux/3
  From41/1 -> Mux/2
  From43/1 -> Mux1/1
  Fourier6/1 -> Gain16/1
  Fourier6/2 -> Sum8/2, Display33/1
  Fourier7/1 -> Gain17/1
  Fourier8/1 -> Gain18/1
  Fourier8/2 -> Sum10/2, Display37/1
  From45/1 -> Mux1/3
  From44/1 -> Mux1/2
  Sum8/1 -> Gain8/1
  Trigonometric Function1/1 -> Display38/1
  Gain8/1 -> Trigonometric Function4/1, Trigonometric Function1/1
  Fourier4/1 -> Gain14/1
  Fourier7/2 -> Sum9/2, Display35/1
  Sum9/1 -> Gain10/1
  Sum10/1 -> Gain12/1
  Mux1/1 -> "Power (3ph, Instantaneous)"/2
  Mux/1 -> "Power (3ph, Instantaneous)"/1
  "Power (3ph, Instantaneous)"/1 -> Display46/1, Scope5/1
  "Power (3ph, Instantaneous)"/2 -> Scope5/2, Display42/1
  Gain13/1 -> Display26/1
  Gain14/1 -> Display28/1
  Gain15/1 -> Display30/1
  Gain16/1 -> Display32/1
  Gain17/1 -> Display34/1
  Gain18/1 -> Display36/1
  Trigonometric Function4/1 -> Display43/1
  Trigonometric Function2/1 -> Display39/1
  Gain10/1 -> Trigonometric Function3/1, Trigonometric Function2/1
  Trigonometric Function3/1 -> Display40/1
  Trigonometric Function5/1 -> Display44/1
  Gain12/1 -> Trigonometric Function5/1, Trigonometric Function6/1
  Trigonometric Function6/1 -> Display45/1
  From5/1 -> Display47/1
  From32/1 -> Display48/1
  From34/1 -> Mux5/1
  From47/1 -> Mux5/3
  From46/1 -> Mux5/2
  From48/1 -> Mux6/1
  From50/1 -> Mux6/3
  From49/1 -> Mux6/2
  Mux6/1 -> "Power (3ph, Instantaneous)1"/2
  Mux5/1 -> "Power (3ph, Instantaneous)1"/1
  "Power (3ph, Instantaneous)1"/1 -> Display50/1, Scope11/1
  "Power (3ph, Instantaneous)1"/2 -> Scope11/2, Display49/1
  From51/1 -> Display51/1
  Bus Selector1/5 -> Goto37/1  "<Stator current is_b (A)>"
  Bus Selector1/4 -> Goto38/1  "<Stator current is_a (A)>"
  Bus Selector1/6 -> Goto36/1  "<Stator current is_c (A)>"
  Bus Selector/6 -> Goto39/1  "<Stator current is_c (A)>"
  Bus Selector/5 -> Goto40/1  "<Stator current is_b (A)>"
  Bus Selector/4 -> Goto41/1  "<Stator current is_a (A)>"
  From52/1 -> Display52/1
  Voltage Measurement/1 -> Goto42/1
  Voltage Measurement1/1 -> Goto43/1
  Voltage Measurement2/1 -> Goto44/1
  Voltage Measurement5/1 -> Goto35/1
  Voltage Measurement4/1 -> Goto34/1
  Voltage Measurement3/1 -> Goto33/1
  Fourier9/1 -> Gain19/1
  Fourier9/2 -> Display54/1
  Gain19/1 -> Display53/1
  From53/1 -> Fourier9/1
  Fourier10/1 -> Gain20/1
  Fourier10/2 -> Display56/1
  Gain20/1 -> Display55/1
  From54/1 -> Fourier10/1
  Fourier12/1 -> Gain21/1
  Fourier12/2 -> Display58/1
  Gain21/1 -> Display57/1
  From55/1 -> Fourier12/1
  Fourier11/1 -> Gain22/1
  Fourier11/2 -> Display60/1
  Gain22/1 -> Display59/1
  From56/1 -> Fourier11/1
  Switch4/1 -> Gain34/1
  PS-Simulink Converter5/1 -> [TorqueShaft]
  Idc_m1/1 -> [IsaM2]
  Idc_m3/1 -> [IsbM2]
  Idc_m4/1 -> [IscM2]
  Vdc_m7/1 -> [VabM2]
  Vdc_m6/1 -> [VbcM2]
  Vdc_m4/1 -> [VcaM2]
  Permanent Magnet Synchronous Machine2/1 -> Bus Selector2/1
  Bus Selector2/3 -> [TeM2]  "<Electromagnetic torque Te (N*m)>"
  Bus Selector2/2 -> [wmM2]  "<Rotor speed wm (rad/s)>"
  Bus Selector2/1 -> [ThetamM2]  "<Rotor angle thetam (rad)>"
  [GateSignalsM2] -> Universal Bridge1/1
  Idc_m5/1 -> [Idc2]
  RMS6/1 -> Display61/1
  Mean4/1 -> Display62/1
  From58/1 -> Mean4/1, RMS6/1
  Sum11/1 -> Relay3/1
  Sum12/1 -> Relay4/1
  Sum13/1 -> Relay5/1
  Data Type Conversion7/1 -> Logical Operator3/1
  Logical Operator3/1 -> Data Type Conversion8/1
  Data Type Conversion8/1 -> Mux7/2
  Data Type Conversion9/1 -> Logical Operator4/1
  Relay4/1 -> Data Type Conversion9/1, Mux7/3
  Logical Operator4/1 -> Data Type Conversion10/1
  Data Type Conversion10/1 -> Mux7/4
  Data Type Conversion11/1 -> Logical Operator5/1
  Relay5/1 -> Data Type Conversion11/1, Mux7/5
  Logical Operator5/1 -> Data Type Conversion12/1
  Data Type Conversion12/1 -> Mux7/6
  Relay3/1 -> Mux7/1, Data Type Conversion7/1
  [VmodCM2] -> Sum13/1
  Triangle Generator1/1 -> Product3/1
  [VdcFilt] -> Product3/2
  Mux7/1 -> [GateSignalsM2]
  Product3/1 -> Sum11/2, Sum12/2, Sum13/2
  [VmodAM2] -> Sum11/1
  [VmodBM2] -> Sum12/1
  Gain23/1 -> [IqrefM1]
  Gain24/1 -> [IqrefM2]
  Constant4/1 -> Gain25/1
  [IsaM2] -> Mux8/1, Scope18/1
  [IsbM2] -> Mux8/2, Scope18/2
  [IscM2] -> Mux8/3, Scope18/3
  [VabM2] -> Scope17/1
  [VbcM2] -> Scope17/2
  [VcaM2] -> Scope17/3
  Mux8/1 -> [IsabcM2]
  [iqM1] -> Scope7/2
  [idM1] -> Scope7/3
  [ThetamModM1] -> Scope7/4
  [VqrefM1] -> Scope9/2
  [VdrefM1] -> Scope9/1
  idref1/1 -> Scope19/1
  [idM1] -> Scope19/2
  [IqrefM1] -> Scope20/1
  [iqM1] -> Scope20/2
  [IsabcM2] -> abc to dq1/1
  Gain26/1 -> abc to dq1/2
  [ThetamM2] -> Gain26/1
  abc to dq1/1 -> Demux2/1
  Demux2/1 -> [idM2]  "id"
  Demux2/2 -> Gain27/1  "iq"
  Demux2/3 -> Terminator1/1  "i0"
  [idM2] -> Sum14/2
  Sum14/1 -> PI iq4/1
  PI iq4/1 -> Saturation3/1
  idref3/1 -> Sum14/1
  [iqM2] -> Sum15/2
  Sum15/1 -> PI iq5/1
  PI iq5/1 -> Saturation4/1
  [IqrefM2] -> Sum15/1
  Saturation4/1 -> [VqrefM2]
  [ThetamM2] -> Gain28/1
  Gain28/1 -> Math Function1/1, dq0 to abc1/2
  Constant8/1 -> Mux9/3
  Mux9/1 -> dq0 to abc1/1
  dq0 to abc1/1 -> Demux3/1
  Demux3/1 -> [VmodAM2]
  Demux3/2 -> [VmodBM2]
  Demux3/3 -> [VmodCM2]
  Constant5/1 -> Math Function1/2
  Math Function1/1 -> [ThetamModM2], Gain29/1
  Gain29/1 -> Scope16/1
  Gain27/1 -> [iqM2]
  Saturation3/1 -> [VdrefM2]
  [VqrefM2] -> Mux9/2
  [VdrefM2] -> Mux9/1
  [IsabcM2] -> Scope21/1
  [iqM2] -> Scope21/2
  [idM2] -> Scope21/3
  [ThetamModM2] -> Scope21/4
  [VqrefM2] -> Scope22/2
  [VdrefM2] -> Scope22/1
  idref4/1 -> Scope23/1
  [idM2] -> Scope23/2
  Clock2/1 -> Switch2/2
  Constant13/1 -> Switch2/1
  Constant16/1 -> Switch2/3
  From92/1 -> Gain30/1
  Gain30/1 -> speed1/2, Sum16/2
  Switch3/1 -> speed1/1, Sum16/1
  Sum16/1 -> PI iq6/1
  PI iq6/1 -> Saturation5/1
  Saturation5/1 -> Gain33/1
  Gain33/1 -> Goto2/1
  Clock3/1 -> Switch3/2
  Constant17/1 -> Switch3/1
  Constant18/1 -> Switch3/3
  Gain31/1 -> Goto69/1
  Gain32/1 -> Goto70/1
  [IqrefM2] -> Scope24/1
  [iqM2] -> Scope24/2
  Clock4/1 -> Switch4/2
  Constant19/1 -> Switch4/1
  Constant20/1 -> Switch4/3
  Gain34/1 -> [Tload], Simulink-PS Converter2/1
  Gain3/1 -> Gain24/1, Gain23/1
  [ThetamM2] -> Scope25/2
  [ThetamM1] -> Scope25/1
  [wmM1] -> Scope26/1
  [wmM2] -> Scope26/2
  [IsabcM1] -> Scope27/3  "iabc1"
  [idM1] -> Bus Creator2/1
  Bus Creator2/1 -> Scope27/1  "id1"
  idref2/1 -> Bus Creator2/2
  Bus Creator1/1 -> Scope27/2  "iq1"
  [iqM1] -> Bus Creator1/1
  [IqrefM1] -> Bus Creator1/2
  [IsabcM2] -> Scope27/6  "iabc2"
  [IqrefM2] -> Bus Creator3/2
  [iqM2] -> Bus Creator3/1
  idref5/1 -> Bus Creator4/2
  [idM2] -> Bus Creator4/1
  Bus Creator4/1 -> Scope27/4  "id2"
  Bus Creator3/1 -> Scope27/5  "iq2"
  [wmM1] -> Bus Creator5/1  "wm"
  Gain35/1 -> Bus Creator5/2  "wref"
  [SpeedRef] -> Gain35/1
  [Tload] -> Gain36/1  "Tload"
  Bus Creator5/1 -> Scope28/1  "rotor speed"
  [TeM1] -> Bus Creator/1  "Te1"
  Bus Creator/1 -> Scope28/2  "Torque"
  [TeM2] -> Bus Creator/2  "Te"
  Gain36/1 -> Bus Creator/3
  Clock1/1 -> Compare To Constant/1
  Compare To Constant/1 -> Ideal Switch/1
  connections:
  Vdc_m5/LConn1 -- Series RLC Branch3/LConn1 -- Vdc_m2/LConn2 -- Ideal Switch/LConn1 -- Idc_m14/RConn1
  Series RLC Branch40/RConn1 -- Ground5/LConn1
  Idc_m14/LConn1 -- Universal Bridge4/LConn1
  Vdc1/RConn1 -- Series RLC Branch20/LConn1
  Idc_m16/LConn1 -- Universal Bridge4/LConn2
  Idc_m17/LConn1 -- Universal Bridge4/LConn3
  Idc_m17/RConn1 -- Permanent Magnet Synchronous Machine/LConn4 -- Vdc_m2/LConn1 -- Vdc_m3/LConn2
  Idc_m16/RConn1 -- Permanent Magnet Synchronous Machine/LConn3 -- Vdc_m3/LConn1 -- Vdc_m5/LConn2
  Universal Bridge4/RConn2 -- Universal Bridge1/RConn2 -- Voltage Measurement6/LConn2 -- Vdc1/LConn1 -- Series RLC Branch40/LConn1 -- Series RLC Branch21/RConn1
  Flexible Shaft/LConn1 -- Ideal Torque Source1/LConn1 -- Solver Configuration/RConn1 -- Inertia/LConn1
  Mechanical Rotational Reference/LConn1 -- Ideal Torque Source1/RConn2
  Simulink-PS Converter1/RConn1 -- Ideal Torque Source1/RConn1
  Ideal Torque Sensor1/LConn1 -- Ideal Torque Sensor3/RConn1 -- Ideal Torque Sensor2/RConn1
  Ideal Torque Sensor1/RConn2 -- PS-Simulink Converter1/LConn1
  Three-Phase Source/RConn2 -- Asynchronous Machine SI Units2/LConn3 -- Voltage Measurement1/LConn1
  Three-Phase Source/RConn3 -- Asynchronous Machine SI Units2/LConn4 -- Voltage Measurement2/LConn1
  Voltage Measurement3/LConn2 -- Voltage Measurement4/LConn2 -- Voltage Measurement5/LConn2 -- Series RLC Branch2/LConn1 -- Series RLC Branch1/LConn1 -- Series RLC Branch/LConn1
  Permanent Magnet Synchronous Machine1/LConn2 -- Series RLC Branch/RConn1 -- Voltage Measurement3/LConn1
  Permanent Magnet Synchronous Machine1/LConn4 -- Series RLC Branch2/RConn1 -- Voltage Measurement5/LConn1
  Permanent Magnet Synchronous Machine1/LConn3 -- Series RLC Branch1/RConn1 -- Voltage Measurement4/LConn1
  Three-Phase Source/RConn1 -- Asynchronous Machine SI Units2/LConn2 -- Voltage Measurement/LConn1
  Ideal Torque Sensor1/RConn1 -- Inertia1/LConn1 -- Flexible Shaft/RConn1
  Ideal Torque Sensor2/LConn1 -- Permanent Magnet Synchronous Machine1/LConn1
  PS-Simulink Converter2/LConn1 -- Ideal Torque Sensor2/RConn2
  PS-Simulink Converter3/LConn1 -- Ideal Torque Sensor3/RConn2
  Asynchronous Machine SI Units2/LConn1 -- Ideal Torque Sensor3/LConn1
  Ground1/LConn1 -- Voltage Measurement2/LConn2 -- Voltage Measurement1/LConn2 -- Voltage Measurement/LConn2
  Inertia2/LConn1 -- Solver Configuration1/RConn1 -- Ideal Torque Source2/LConn1 -- Flexible Shaft1/LConn1
  Inertia3/LConn1 -- Flexible Shaft1/RConn1 -- Ideal Torque Sensor5/RConn1
  Simulink-PS Converter2/RConn1 -- Ideal Torque Source2/RConn1
  PS-Simulink Converter5/LConn1 -- Ideal Torque Sensor5/RConn2
  Mechanical Rotational Reference1/LConn1 -- Ideal Torque Source2/RConn2
  Idc_m1/RConn1 -- Vdc_m7/LConn1 -- Vdc_m4/LConn2 -- Permanent Magnet Synchronous Machine2/LConn2
  Vdc_m6/LConn2 -- Idc_m4/RConn1 -- Vdc_m4/LConn1 -- Permanent Magnet Synchronous Machine2/LConn4
  Vdc_m6/LConn1 -- Idc_m3/RConn1 -- Vdc_m7/LConn2 -- Permanent Magnet Synchronous Machine2/LConn3
  Idc_m1/LConn1 -- Universal Bridge1/LConn1
  Idc_m3/LConn1 -- Universal Bridge1/LConn2
  Idc_m4/LConn1 -- Universal Bridge1/LConn3
  Current Measurement1/RConn1 -- Universal Bridge4/RConn1
  Universal Bridge1/RConn1 -- Idc_m5/RConn1
  Current Measurement/LConn1 -- Series RLC Branch20/RConn1
  Current Measurement/RConn1 -- Idc_m5/LConn1 -- Current Measurement1/LConn1 -- Voltage Measurement6/LConn1 -- Series RLC Branch21/LConn1
  Permanent Magnet Synchronous Machine/LConn1 -- Permanent Magnet Synchronous Machine2/LConn1 -- Ideal Torque Sensor5/LConn1
  Ideal Switch/RConn1 -- Series RLC Branch3/RConn1 -- Permanent Magnet Synchronous Machine/LConn2
